simulink library "dclink_for_two_levels"  (R2025b)
settings: Solver=VariableStepAuto  StartTime=0.0  StopTime=10.0  RelTol=1e-3
undefined symbols (not defined in the file): Vbattery_nom
libraries: fl_lib x16, nesl_utility x7
settings Model: Creator=dbagn  LastModifiedBy=ltnbda

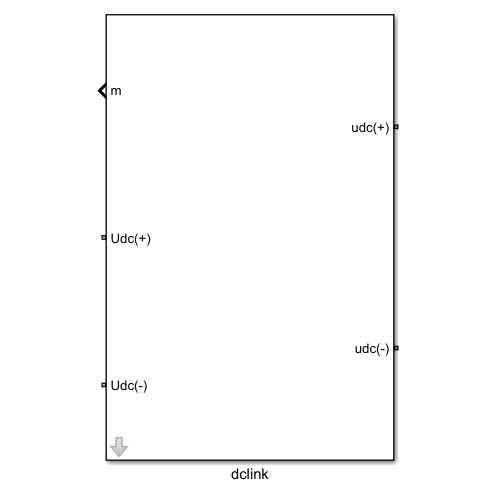
[thumbnail: Simulink's stored preview of the top-level diagram]
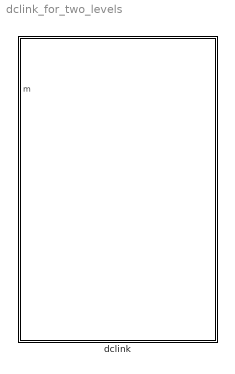
== system dclink_for_two_levels ==
  dclink : Subsystem  mask{Cdc=7.2e-3, Rudc_measure=107e3, Vdc_scale=1070}
      mask prompts: Cdc "Cdc1"

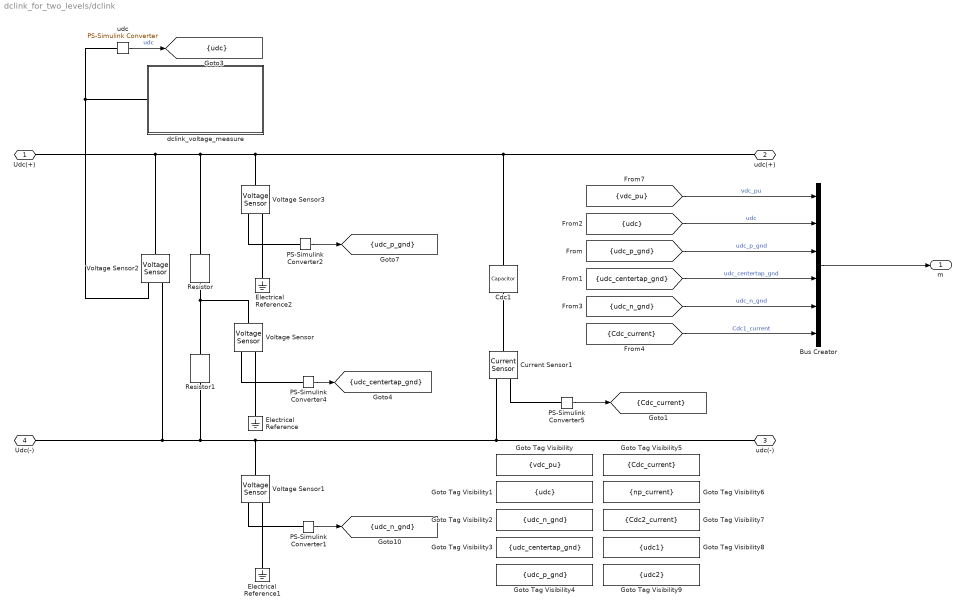
== system dclink_for_two_levels/dclink ==
  Bus Creator : BusCreator  Inputs=6
  Cdc1 : fl_lib/Electrical/Electrical Elements/Capacitor  c=Cdc F  r=2e-3 Ohm  g=0 1/Ohm  i_specify=on  i_priority=None  i=0 A  i_nominal_specify=off  i_nominal_value=1  i_nominal_unit=A  v_specify=off  v_priority=High  v=Vbattery_nom/2 V  v_nominal_specify=off  v_nominal_value=1  v_nominal_unit=V  vc_specify=off  vc_priority=High  vc=0 V  vc_nominal_specify=off  vc_nominal_value=1  vc_nominal_unit=V
  Current Sensor1 : fl_lib/Electrical/Electrical Sensors/Current Sensor
  Electrical Reference : fl_lib/Electrical/Electrical Elements/Electrical Reference
  Electrical Reference1 : fl_lib/Electrical/Electrical Elements/Electrical Reference
  Electrical Reference2 : fl_lib/Electrical/Electrical Elements/Electrical Reference
  Goto Tag Visibility : GotoTagVisibility  GotoTag=vdc_pu
  Goto Tag Visibility1 : GotoTagVisibility  GotoTag=udc
  Goto Tag Visibility2 : GotoTagVisibility  GotoTag=udc_n_gnd
  Goto Tag Visibility3 : GotoTagVisibility  GotoTag=udc_centertap_gnd
  Goto Tag Visibility4 : GotoTagVisibility  GotoTag=udc_p_gnd
  Goto Tag Visibility5 : GotoTagVisibility  GotoTag=Cdc_current
  Goto Tag Visibility6 : GotoTagVisibility  GotoTag=np_current
  Goto Tag Visibility7 : GotoTagVisibility  GotoTag=Cdc2_current
  Goto Tag Visibility8 : GotoTagVisibility  GotoTag=udc1
  Goto Tag Visibility9 : GotoTagVisibility  GotoTag=udc2
  PS-Simulink Converter1 : nesl_utility/PS-Simulink Converter  PhysicalDomain=network_engine_domain  SubClassName=ps_output  LeftPortType=input  RightPortType=output  PseudoPeriodic=off  Frequencies=[]  VectorFormat=1-D array  Unit=V  AffineConversion=on
  PS-Simulink Converter2 : nesl_utility/PS-Simulink Converter  PhysicalDomain=network_engine_domain  SubClassName=ps_output  LeftPortType=input  RightPortType=output  PseudoPeriodic=off  Frequencies=[]  VectorFormat=1-D array  Unit=V  AffineConversion=on
  PS-Simulink Converter4 : nesl_utility/PS-Simulink Converter  PhysicalDomain=network_engine_domain  SubClassName=ps_output  LeftPortType=input  RightPortType=output  PseudoPeriodic=off  Frequencies=[]  VectorFormat=1-D array  Unit=V  AffineConversion=on
  PS-Simulink Converter5 : nesl_utility/PS-Simulink Converter  PhysicalDomain=network_engine_domain  SubClassName=ps_output  LeftPortType=input  RightPortType=output  PseudoPeriodic=off  Frequencies=[]  VectorFormat=1-D array  Unit=A  AffineConversion=on
  Resistor : fl_lib/Electrical/Electrical Elements/Resistor  R=1e6 Ohm  i_specify=off  i_priority=None  i=0 A  i_nominal_specify=off  i_nominal_value=1  i_nominal_unit=A  v_specify=off  v_priority=None  v=0 V  v_nominal_specify=off  v_nominal_value=1  v_nominal_unit=V
  Resistor1 : fl_lib/Electrical/Electrical Elements/Resistor  R=1e6 Ohm  i_specify=off  i_priority=None  i=0 A  i_nominal_specify=off  i_nominal_value=1  i_nominal_unit=A  v_specify=off  v_priority=None  v=0 V  v_nominal_specify=off  v_nominal_value=1  v_nominal_unit=V
  Voltage Sensor{,1..3} (4 alike) : fl_lib/Electrical/Electrical Sensors/Voltage Sensor
  dclink_voltage_measure : Subsystem
  udc : nesl_utility/PS-Simulink Converter  PhysicalDomain=network_engine_domain  SubClassName=ps_output  LeftPortType=input  RightPortType=output  PseudoPeriodic=off  Frequencies=[]  VectorFormat=1-D array  Unit=V  AffineConversion=on
  Udc(+) : PMIOPort  Side=Right
  udc(+) : PMIOPort  Port=2  Side=Left
  udc(-) : PMIOPort  Port=3  Side=Left
  Udc(-) : PMIOPort  Port=4  Side=Right
  m : Outport
  tag scope: Cdc_current=scoped, udc=scoped, udc_centertap_gnd=scoped, udc_n_gnd=scoped, udc_p_gnd=scoped
  wires:
  PS-Simulink Converter2/1 -> [udc_p_gnd]
  PS-Simulink Converter1/1 -> [udc_n_gnd]
  udc/1 -> [udc]  "udc"
  PS-Simulink Converter5/1 -> [Cdc_current]
  PS-Simulink Converter4/1 -> [udc_centertap_gnd]
  [vdc_pu] -> Bus Creator/1  "vdc_pu"
  [udc] -> Bus Creator/2  "udc"
  [udc_p_gnd] -> Bus Creator/3  "udc_p_gnd"
  [udc_centertap_gnd] -> Bus Creator/4  "udc_centertap_gnd"
  [udc_n_gnd] -> Bus Creator/5  "udc_n_gnd"
  [Cdc_current] -> Bus Creator/6  "Cdc1_current"
  Bus Creator/1 -> m/1
  connections:
  Voltage Sensor/RConn2 -- Electrical Reference/LConn1
  Voltage Sensor3/RConn2 -- Electrical Reference2/LConn1
  Current Sensor1/RConn2 -- udc(-)/RConn1 -- Voltage Sensor1/LConn1 -- Voltage Sensor2/RConn2 -- Udc(-)/RConn1 -- Resistor1/RConn1
  Voltage Sensor/RConn1 -- PS-Simulink Converter4/LConn1
  Voltage Sensor2/RConn1 -- udc/LConn1 -- dclink_voltage_measure/LConn1
  PS-Simulink Converter2/LConn1 -- Voltage Sensor3/RConn1
  Voltage Sensor1/RConn2 -- Electrical Reference1/LConn1
  Cdc1/LConn1 -- udc(+)/RConn1 -- Voltage Sensor3/LConn1 -- Resistor/LConn1 -- Udc(+)/RConn1 -- Voltage Sensor2/LConn1
  Resistor1/LConn1 -- Voltage Sensor/LConn1 -- Resistor/RConn1
  PS-Simulink Converter1/LConn1 -- Voltage Sensor1/RConn1
  Current Sensor1/LConn1 -- Cdc1/RConn1
  Current Sensor1/RConn1 -- PS-Simulink Converter5/LConn1

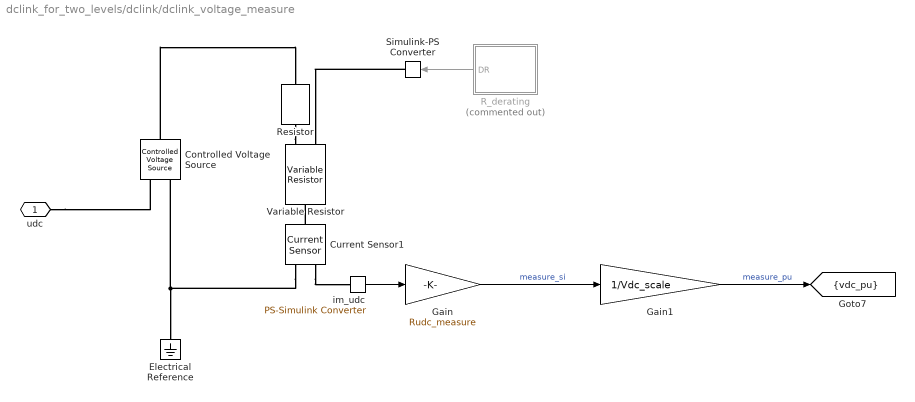
== system dclink_for_two_levels/dclink/dclink_voltage_measure ==
  Controlled Voltage Source : fl_lib/Electrical/Electrical Sources/Controlled Voltage Source
  Current Sensor1 : fl_lib/Electrical/Electrical Sensors/Current Sensor
  Electrical Reference : fl_lib/Electrical/Electrical Elements/Electrical Reference
  Gain : Gain  Gain=Rudc_measure
  Gain1 : Gain  Gain=1/Vdc_scale
  R_derating : Subsystem  Commented=on
  Resistor : fl_lib/Electrical/Electrical Elements/Resistor  R=Rudc_measure Ohm  i_specify=off  i_priority=None  i=0 A  i_nominal_specify=off  i_nominal_value=1  i_nominal_unit=A  v_specify=off  v_priority=None  v=0 V  v_nominal_specify=off  v_nominal_value=1  v_nominal_unit=V
  Simulink-PS Converter : nesl_utility/Simulink-PS Converter  PhysicalDomain=network_engine_domain  SubClassName=ps_input  LeftPortType=input  RightPortType=output  PseudoPeriodic=off  Frequencies=[]  NoiseDistribution=none  NoiseParameters=[]  Unit=Ohm  AffineConversion=off  FilteringAndDerivatives=provide  SimscapeFilterOrder=1  InputFilterTimeConstant=0.001  UdotUserProvided=0
  Variable Resistor : fl_lib/Electrical/Electrical Elements/Variable Resistor  Rmin=0 Ohm  thermalEnable=false  thermal_mass=1 J/K  i_specify=off  i_priority=None  i=0 A  i_nominal_specify=off  i_nominal_value=1  i_nominal_unit=A  v_specify=off  v_priority=None  v=0 V  v_nominal_specify=off  v_nominal_value=1  v_nominal_unit=V  T_specify=off  T_priority=None  T=300 K  T_nominal_specify=off  T_nominal_value=1  T_nominal_unit=K
  im_udc : nesl_utility/PS-Simulink Converter  PhysicalDomain=network_engine_domain  SubClassName=ps_output  LeftPortType=input  RightPortType=output  PseudoPeriodic=off  Frequencies=[]  VectorFormat=1-D array  Unit=A  AffineConversion=on
  udc : PMIOPort  Side=Left
  tag scope: vdc_pu=scoped
  wires:
  Gain/1 -> Gain1/1  "measure_si"
  im_udc/1 -> Gain/1
  Gain1/1 -> [vdc_pu]  "measure_pu"
  R_derating/1(DR) -> Simulink-PS Converter/1
  connections:
  udc/RConn1 -- Controlled Voltage Source/RConn1
  Resistor/RConn1 -- Variable Resistor/LConn2
  Current Sensor1/RConn1 -- im_udc/LConn1
  Current Sensor1/RConn2 -- Electrical Reference/LConn1 -- Controlled Voltage Source/RConn2
  Current Sensor1/LConn1 -- Variable Resistor/RConn1
  Simulink-PS Converter/RConn1 -- Variable Resistor/LConn1
  Controlled Voltage Source/LConn1 -- Resistor/LConn1

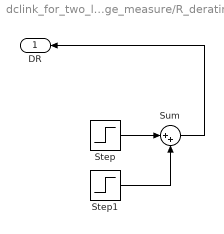
== system dclink_for_two_levels/dclink/dclink_voltage_measure/R_derating ==
  Step : Step  After=107.4e3/2  SampleTime=0
  Step1 : Step  Time=1.1  After=-107.4e3/2  SampleTime=0
  Sum : Sum  Inputs=|++
  DR : Outport
  wires:
  Step1/1 -> Sum/2
  Step/1 -> Sum/1
  Sum/1 -> DR/1
